simulink model "SVPWM_model"  (R2021b)
settings: Solver=ode3  StartTime=0.0  StopTime=0.3  FixedStep=1e-5  RelTol=1e-3
libraries: simulink x4, spspowerguiLib x1
settings Model: Creator=zyh  LastModifiedBy=zyh
settings SolverCC: AlgebraicLoopSolver=TrustRegion
settings DataIOCC: ReturnWorkspaceOutputs=off
settings DebuggingCC: MaskedZcDiagnostic=none  IgnoredZcDiagnostic=none  SFMachineParentedDataDiag=warning  ArithmeticOperatorsInVariantConditions=warning
settings SFSimCC: CustomCodeUndefinedFunction=UseInterfaceOnly

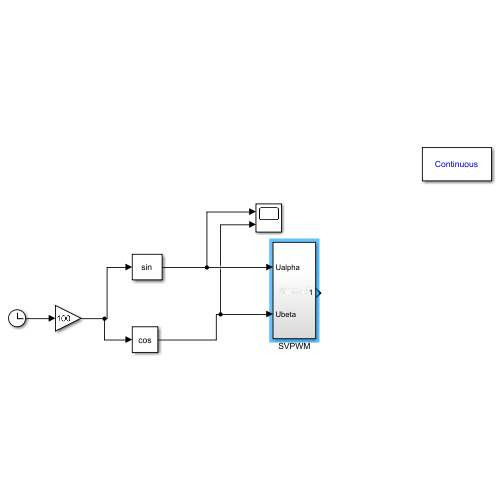
[thumbnail: Simulink's stored preview of the top-level diagram]
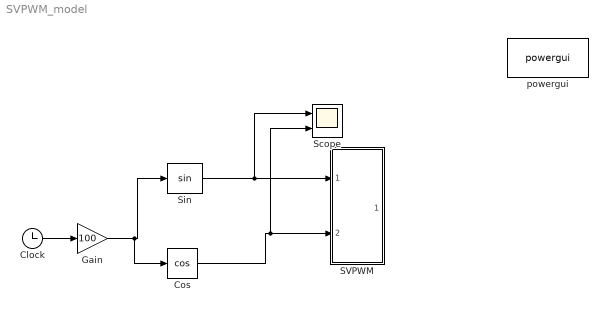
== system SVPWM_model ==
  Clock : Clock
  Cos : Trigonometry  Operator=cos
  Gain : Gain  Gain=100
  SVPWM : Subsystem
  Scope : Scope  NumInputPorts=2
  Sin : Trigonometry
  powergui : spspowerguiLib/powergui  Priority=1  SimulationMode=Continuous  SampleTime=1e-6  frequency=60  Iterations=50  frequencyindice=0  Pbase=100e6  ErrMax=1e-4  UnitsV=kV  UnitsW=MW  buscounter=0  FunctionMessages=off  echomessages=off  EnableUseOfTLC=off  CurrentSourceSwitches=off  DisableSnubberDevices=off  DisableRonSwitches=off  DisableVfSwitches=off  DisplayEquations=off  AutomaticDiscreteSolvers=off  SolverType=Tustin/Backward Euler (TBE)  Interpol=off  ExternalGateDelay=off  methode=off  Ts=100  x0status=blocks  SPID=on  SwTol=0  HookPort=off  NonlinearTolerance=1e-4  nMaxIteration=100  ContinueOnMaxIteration=off  RestoreLinks=warning  ResistiveCurrentMeasurement=off  Frange=[0:2:500]  Ylog=off  Xlog=on  ShowGrid=off  save=off  variable=ZData  structure=0  ZoomFFT=off  StartTime=0.0  cycles=1  DisplayStyle=1  fundamental=60  FreqAxis=off  MaxFrequency=1000  frequencyindicesteady=1  RmsSteady=1  display=off
  wires:
  Clock/1 -> Gain/1
  Gain/1 -> Cos/1, Sin/1
  Sin/1 -> Scope/1, SVPWM/1(Ualpha)
  Cos/1 -> Scope/2, SVPWM/2(Ubeta)

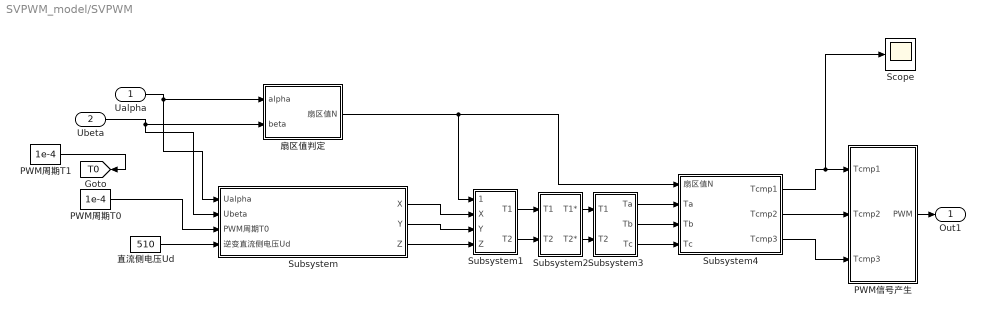
== system SVPWM_model/SVPWM ==
  Ualpha : Inport
  Ubeta : Inport  Port=2
  PWM信号产生 : Subsystem
  PWM周期T0 : Constant  Value=1e-4
  PWM周期T1 : Constant  Value=1e-4
  Scope : Scope
  Subsystem : Subsystem
  Subsystem1 : Subsystem
  Subsystem2 : Subsystem
  Subsystem3 : Subsystem
  Subsystem4 : Subsystem
  扇区值判定 : Subsystem
  直流侧电压Ud : Constant  Value=510
  Out1 : Outport  VectorParamsAs1DForOutWhenUnconnected=off
  tag scope: T0=global
  wires:
  Subsystem2/2(T2*) -> Subsystem3/2(T2)
  Subsystem1/2(T2) -> Subsystem2/2(T2)
  Subsystem4/1(Tcmp1) -> PWM信号产生/1(Tcmp1), Scope/1
  Subsystem3/2(Tb) -> Subsystem4/3(Tb)
  直流侧电压Ud/1 -> Subsystem/4(逆变直流侧电压Ud)
  Ualpha/1 -> 扇区值判定/1(alpha), Subsystem/1(Ualpha)
  Subsystem/3(Z) -> Subsystem1/4(Z)
  Subsystem3/3(Tc) -> Subsystem4/4(Tc)
  PWM信号产生/1(PWM) -> Out1/1
  Subsystem3/1(Ta) -> Subsystem4/2(Ta)
  PWM周期T0/1 -> Subsystem/3(PWM周期T0)
  Subsystem4/2(Tcmp2) -> PWM信号产生/2(Tcmp2)
  扇区值判定/1(扇区值N) -> Subsystem4/1(扇区值N), Subsystem1/1(扇区值N)
  Subsystem4/3(Tcmp3) -> PWM信号产生/3(Tcmp3)
  Subsystem/2(Y) -> Subsystem1/3(Y)
  Ubeta/1 -> 扇区值判定/2(beta), Subsystem/2(Ubeta)
  Subsystem/1(X) -> Subsystem1/2(X)
  Subsystem1/1(T1) -> Subsystem2/1(T1)
  Subsystem2/1(T1*) -> Subsystem3/1(T1)
  PWM周期T1/1 -> [T0]

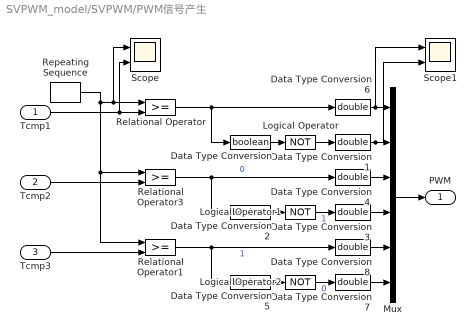
== system SVPWM_model/SVPWM/PWM信号产生 ==
  Tcmp1 : Inport
  Tcmp2 : Inport  Port=2
  Tcmp3 : Inport  Port=3
  Data Type Conversion : DataTypeConversion  OutDataTypeStr=boolean
  Data Type Conversion{1,3..4,6..8} (6 alike) : DataTypeConversion  OutDataTypeStr=double
  Data Type Conversion2 : DataTypeConversion  OutDataTypeStr=boolean
  Data Type Conversion5 : DataTypeConversion  OutDataTypeStr=boolean
  Logical Operator : Logic  Operator=NOT  AllPortsSameDT=off  OutDataTypeStr=boolean
  Logical Operator1 : Logic  Operator=NOT  AllPortsSameDT=off  OutDataTypeStr=boolean
  Logical Operator2 : Logic  Operator=NOT  AllPortsSameDT=off  OutDataTypeStr=boolean
  Mux : Mux  Inputs=6
  Relational Operator : RelationalOperator  OutDataTypeStr=boolean  RndMeth=Nearest
  Relational Operator1 : RelationalOperator  OutDataTypeStr=boolean  RndMeth=Nearest
  Relational Operator3 : RelationalOperator  OutDataTypeStr=boolean  RndMeth=Nearest
  Repeating Sequence : simulink/Sources/Repeating Sequence  rep_seq_t=[0 1e-4 2e-4]  rep_seq_y=[0 1.3e-6 0]
  Scope : Scope  NumInputPorts=2
  Scope1 : Scope  NumInputPorts=2
  PWM : Outport  VectorParamsAs1DForOutWhenUnconnected=off
  wires:
  Data Type Conversion6/1 -> Mux/1, Scope1/1
  Mux/1 -> PWM/1
  Data Type Conversion7/1 -> Mux/6
  Data Type Conversion8/1 -> Mux/5
  Data Type Conversion3/1 -> Mux/4
  Data Type Conversion4/1 -> Mux/3
  Data Type Conversion1/1 -> Mux/2, Scope1/2
  Tcmp3/1 -> Relational Operator1/2
  Tcmp2/1 -> Relational Operator3/2
  Tcmp1/1 -> Relational Operator/2, Scope/2
  Repeating Sequence/1 -> Relational Operator/1, Scope/1, Relational Operator3/1, Relational Operator1/1
  Logical Operator2/1 -> Data Type Conversion7/1  "0"
  Data Type Conversion5/1 -> Logical Operator2/1
  Relational Operator1/1 -> Data Type Conversion5/1, Data Type Conversion8/1  "1"
  Data Type Conversion2/1 -> Logical Operator1/1
  Relational Operator3/1 -> Data Type Conversion2/1, Data Type Conversion4/1  "0"
  Logical Operator1/1 -> Data Type Conversion3/1  "1"
  Relational Operator/1 -> Data Type Conversion/1, Data Type Conversion6/1
  Logical Operator/1 -> Data Type Conversion1/1
  Data Type Conversion/1 -> Logical Operator/1

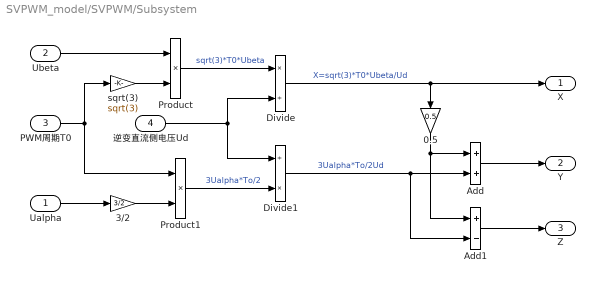
== system SVPWM_model/SVPWM/Subsystem ==
  Ualpha : Inport
  Ubeta : Inport  Port=2
  PWM周期T0 : Inport  Port=3
  逆变直流侧电压Ud : Inport  Port=4
  0.5 : Gain  Gain=0.5
  3/2 : Gain  Gain=3/2
  Add : Sum
  Add1 : Sum  Inputs=+-
  Divide : Product  Inputs=*/
  Divide1 : Product  Inputs=/*
  Product : Product
  Product1 : Product
  "sqrt(3) " : Gain  Gain=sqrt(3)
  X : Outport  VectorParamsAs1DForOutWhenUnconnected=off
  Y : Outport  Port=2  VectorParamsAs1DForOutWhenUnconnected=off
  Z : Outport  Port=3  VectorParamsAs1DForOutWhenUnconnected=off
  wires:
  Product/1 -> Divide/1  "sqrt(3)*T0*Ubeta"
  Add1/1 -> Z/1
  Divide1/1 -> Add/2, Add1/2  "3Ualpha*To/2Ud"
  Ubeta/1 -> Product/1
  Ualpha/1 -> 3/2/1
  Add/1 -> Y/1
  Product1/1 -> Divide1/2  "3Ualpha*To/2"
  3/2/1 -> Product1/2
  "sqrt(3) "/1 -> Product/2
  PWM周期T0/1 -> Product1/1, "sqrt(3) "/1
  0.5/1 -> Add1/1, Add/1
  逆变直流侧电压Ud/1 -> Divide/2, Divide1/1
  Divide/1 -> 0.5/1, X/1  "X=sqrt(3)*T0*Ubeta/Ud"

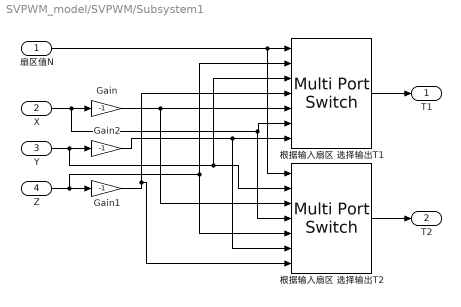
== system SVPWM_model/SVPWM/Subsystem1 ==
  扇区值N : Inport
  X : Inport  Port=2
  Y : Inport  Port=3
  Z : Inport  Port=4
  Gain : Gain  Gain=-1
  Gain1 : Gain  Gain=-1
  Gain2 : Gain  Gain=-1
  根据输入扇区 选择输出T1 : MultiPortSwitch  Inputs=6  DiagnosticForDefault=None
  根据输入扇区 选择输出T2 : MultiPortSwitch  Inputs=6  DiagnosticForDefault=None
  T1 : Outport  VectorParamsAs1DForOutWhenUnconnected=off
  T2 : Outport  Port=2  VectorParamsAs1DForOutWhenUnconnected=off
  wires:
  扇区值N/1 -> 根据输入扇区 选择输出T1/1, 根据输入扇区 选择输出T2/1
  Gain2/1 -> 根据输入扇区 选择输出T1/7, 根据输入扇区 选择输出T2/6
  根据输入扇区 选择输出T2/1 -> T2/1
  根据输入扇区 选择输出T1/1 -> T1/1
  Gain/1 -> 根据输入扇区 选择输出T2/3, 根据输入扇区 选择输出T1/5
  Gain1/1 -> 根据输入扇区 选择输出T1/4, 根据输入扇区 选择输出T2/7
  Z/1 -> Gain1/1, 根据输入扇区 选择输出T1/2, 根据输入扇区 选择输出T2/5
  Y/1 -> Gain2/1, 根据输入扇区 选择输出T2/2, 根据输入扇区 选择输出T1/3
  X/1 -> Gain/1, 根据输入扇区 选择输出T1/6, 根据输入扇区 选择输出T2/4

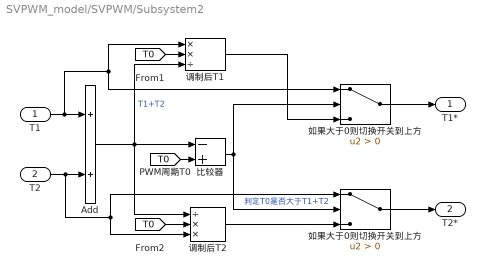
== system SVPWM_model/SVPWM/Subsystem2 ==
  T1 : Inport
  T2 : Inport  Port=2
  Add : Sum
  如果大于0则切换开关到上方 : Switch  Criteria=u2 > Threshold
  "如果大于0则切换开关到上方 " : Switch  Criteria=u2 > Threshold
  比较器 : Sum  Inputs=-+
  调制后T1 : Product  Inputs=**/
  调制后T2 : Product  Inputs=/**
  T1* : Outport  VectorParamsAs1DForOutWhenUnconnected=off
  T2* : Outport  Port=2  VectorParamsAs1DForOutWhenUnconnected=off
  wires:
  T2/1 -> Add/2, 调制后T2/3, "如果大于0则切换开关到上方 "/1
  调制后T2/1 -> "如果大于0则切换开关到上方 "/3
  如果大于0则切换开关到上方/1 -> T1*/1
  [T0] -> 比较器/2
  T1/1 -> Add/1, 调制后T1/1, 如果大于0则切换开关到上方/1
  [T0] -> 调制后T1/2
  Add/1 -> 调制后T1/3, 比较器/1, 调制后T2/1  "T1+T2"
  [T0] -> 调制后T2/2
  比较器/1 -> 如果大于0则切换开关到上方/2, "如果大于0则切换开关到上方 "/2  "判定T0是否大于T1+T2"
  "如果大于0则切换开关到上方 "/1 -> T2*/1
  调制后T1/1 -> 如果大于0则切换开关到上方/3

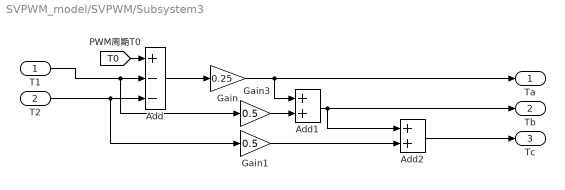
== system SVPWM_model/SVPWM/Subsystem3 ==
  T1 : Inport
  T2 : Inport  Port=2
  Add : Sum  Inputs=+--
  Add1 : Sum
  Add2 : Sum
  Gain : Gain  Gain=0.25
  Gain1 : Gain  Gain=0.5
  Gain3 : Gain  Gain=0.5
  Ta : Outport  VectorParamsAs1DForOutWhenUnconnected=off
  Tb : Outport  Port=2  VectorParamsAs1DForOutWhenUnconnected=off
  Tc : Outport  Port=3  VectorParamsAs1DForOutWhenUnconnected=off
  wires:
  T2/1 -> Add/3, Gain1/1
  Gain/1 -> Add1/1, Ta/1
  Gain1/1 -> Add2/2
  Gain3/1 -> Add1/2
  Add1/1 -> Add2/1, Tb/1
  T1/1 -> Add/2, Gain3/1
  [T0] -> Add/1
  Add/1 -> Gain/1
  Add2/1 -> Tc/1

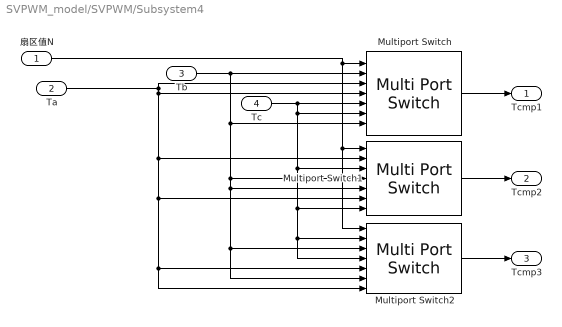
== system SVPWM_model/SVPWM/Subsystem4 ==
  扇区值N : Inport
  Ta : Inport  Port=2
  Tb : Inport  Port=3
  Tc : Inport  Port=4
  Multiport Switch : MultiPortSwitch  Inputs=6  DiagnosticForDefault=None  OutDataTypeStr=double
  Multiport Switch1 : MultiPortSwitch  Inputs=6  DiagnosticForDefault=None  OutDataTypeStr=double
  Multiport Switch2 : MultiPortSwitch  Inputs=6  DiagnosticForDefault=None  OutDataTypeStr=double
  Tcmp1 : Outport  VectorParamsAs1DForOutWhenUnconnected=off
  Tcmp2 : Outport  Port=2  VectorParamsAs1DForOutWhenUnconnected=off
  Tcmp3 : Outport  Port=3  VectorParamsAs1DForOutWhenUnconnected=off
  wires:
  Multiport Switch2/1 -> Tcmp3/1
  Tc/1 -> Multiport Switch/5, Multiport Switch/6, Multiport Switch1/3, Multiport Switch2/4, Multiport Switch2/2, Multiport Switch1/7
  Multiport Switch1/1 -> Tcmp2/1
  Ta/1 -> Multiport Switch1/2, Multiport Switch1/6, Multiport Switch2/5, Multiport Switch2/7, Multiport Switch/4, Multiport Switch/3
  Multiport Switch/1 -> Tcmp1/1
  Tb/1 -> Multiport Switch/2, Multiport Switch/7, Multiport Switch1/4, Multiport Switch1/5, Multiport Switch2/3, Multiport Switch2/6
  扇区值N/1 -> Multiport Switch/1, Multiport Switch1/1, Multiport Switch2/1

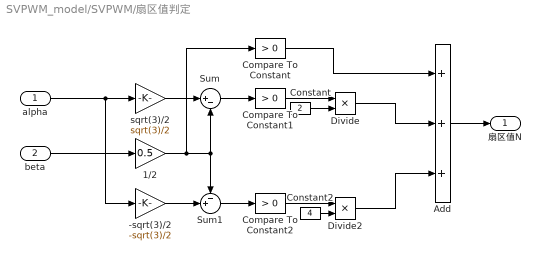
== system SVPWM_model/SVPWM/扇区值判定 ==
  alpha : Inport
  beta : Inport  Port=2
  -sqrt(3)/2 : Gain  Gain=-sqrt(3)/2
  1/2 : Gain  Gain=0.5
  "Add " : Sum  Inputs=+++
  Compare To Constant : simulink/Logic and Bit Operations/Compare To Constant  relop=>  const=0  OutDataTypeStr=boolean
  Compare To Constant1 : simulink/Logic and Bit Operations/Compare To Constant  relop=>  const=0  OutDataTypeStr=boolean
  Compare To Constant2 : simulink/Logic and Bit Operations/Compare To Constant  relop=>  const=0  OutDataTypeStr=boolean
  Constant : Constant  Value=2
  Constant2 : Constant  Value=4
  Divide : Product  Inputs=**
  Divide2 : Product  Inputs=**
  Sum : Sum  Inputs=|+-
  Sum1 : Sum  Inputs=-+|
  sqrt(3)/2 : Gain  Gain=sqrt(3)/2
  扇区值N : Outport  VectorParamsAs1DForOutWhenUnconnected=off
  wires:
  alpha/1 -> sqrt(3)/2/1, -sqrt(3)/2/1
  Constant/1 -> Divide/2
  Divide/1 -> "Add "/2
  Compare To Constant1/1 -> Divide/1
  Compare To Constant/1 -> "Add "/1
  sqrt(3)/2/1 -> Sum/1
  beta/1 -> 1/2/1
  Compare To Constant2/1 -> Divide2/1
  "Add "/1 -> 扇区值N/1
  1/2/1 -> Compare To Constant/1, Sum/2, Sum1/1
  Constant2/1 -> Divide2/2
  Sum1/1 -> Compare To Constant2/1
  -sqrt(3)/2/1 -> Sum1/2
  Sum/1 -> Compare To Constant1/1
  Divide2/1 -> "Add "/3
